simulink model "Alpha_Beta_sim"  (R2019b)
settings: Solver=VariableStepAuto  StartTime=0.0  StopTime=t_sim  FixedStep=1e-6  RelTol=1e-8  AbsTol=1e-8
values from neighbouring files (symbols this model uses):
  alphaCond = 0    [MarsTetherDynamics.m]
  betaCond = 0    [MarsTetherDynamics.m]
  dAlphaCond = 0    [MarsTetherDynamics.m]
  dBetaCond = 0    [MarsTetherDynamics.m]
  Dtheta = v/ (lt+r_hub)    (= 0.00487620861696)    [MarsTetherDynamics.m]
  g_mars = 3.71    [MarsTetherDynamics.m]
  lt = (v^2)/gamma_max    (= 824771.150189)    [MarsTetherDynamics.m]
  omega = 2*pi/T_mars    (= 7.0776580899e-05)    [MarsTetherDynamics.m]
  phi = 18.65 *pi/180    (= 0.325503905497)    [MarsTetherDynamics.m]
  r_hub = 50    [MarsTetherDynamics.m]
settings Model: Creator=valentinrichard  LastModifiedBy=valentinrichard

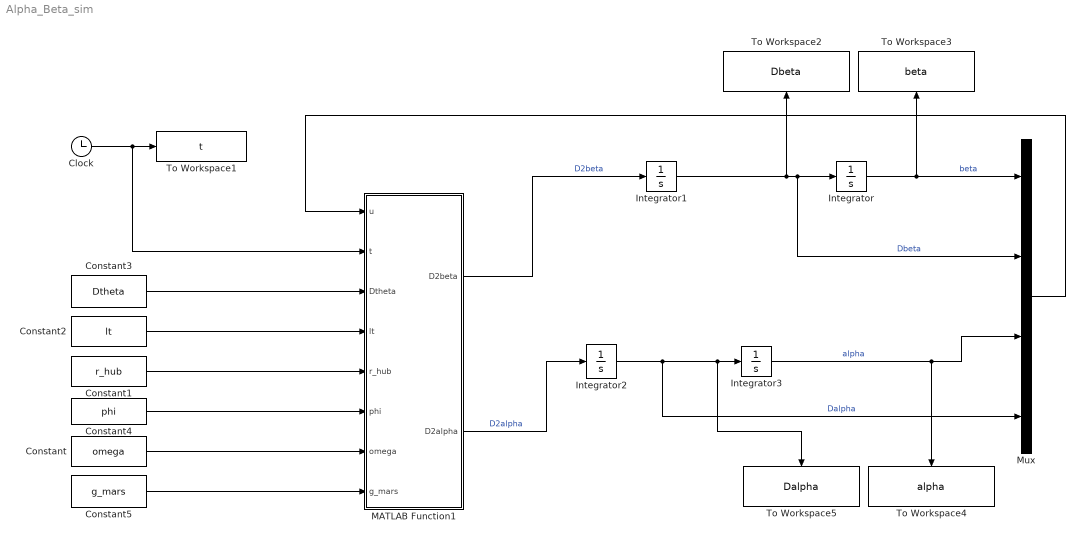
== system Alpha_Beta_sim ==
  Clock : Clock
  Constant : Constant  Value=omega
  Constant1 : Constant  Value=r_hub
  Constant2 : Constant  Value=lt
  Constant3 : Constant  Value=Dtheta
  Constant4 : Constant  Value=phi
  Constant5 : Constant  Value=g_mars
  Integrator : Integrator  InitialCondition=betaCond
  Integrator1 : Integrator  InitialCondition=dBetaCond
  Integrator2 : Integrator  InitialCondition=dAlphaCond
  Integrator3 : Integrator  InitialCondition=alphaCond
  MATLAB Function1 : MATLAB Function  TreatAsAtomicUnit=on
  Mux : Mux
  To Workspace1 : ToWorkspace  VariableName=t  SampleTime=-1
  To Workspace2 : ToWorkspace  VariableName=Dbeta  SampleTime=-1
  To Workspace3 : ToWorkspace  VariableName=beta  SampleTime=-1
  To Workspace4 : ToWorkspace  VariableName=alpha  SampleTime=-1
  To Workspace5 : ToWorkspace  VariableName=Dalpha  SampleTime=-1
  wires:
  Integrator2/1 -> To Workspace5/1, Integrator3/1, Mux/4  "Dalpha"
  Integrator1/1 -> To Workspace2/1, Mux/2, Integrator/1  "Dbeta"
  Integrator/1 -> To Workspace3/1, Mux/1  "beta"
  Integrator3/1 -> To Workspace4/1, Mux/3  "alpha"
  Mux/1 -> MATLAB Function1/1(u)
  MATLAB Function1/2(D2alpha) -> Integrator2/1  "D2alpha"
  MATLAB Function1/1(D2beta) -> Integrator1/1  "D2beta"
  Clock/1 -> MATLAB Function1/2(t), To Workspace1/1
  Constant3/1 -> MATLAB Function1/3(Dtheta)
  Constant2/1 -> MATLAB Function1/4(lt)
  Constant1/1 -> MATLAB Function1/5(r_hub)
  Constant4/1 -> MATLAB Function1/6(phi)
  Constant/1 -> MATLAB Function1/7(omega)
  Constant5/1 -> MATLAB Function1/8(g_mars)

== matlab function Alpha_Beta_sim/MATLAB Function1 ==
  data: D2beta output; u input; D2alpha output; t input; Dtheta input; lt input; r_hub input; phi input; omega input; g_mars input
function [ D2beta, D2alpha ] = ode(u,t,Dtheta,lt,r_hub,phi,omega,g_mars)
% Differential equation for Beta
%   beta = beta
%   Dbeta = d/dt (beta)
%   alpha = alpha 
%   Dalpha = d/dt (alpha)

beta = u(1);
Dbeta = u(2);
alpha = u(3);
Dalpha = u(4);


D2alpha = -2*Dbeta*tan(beta)*(Dtheta-Dalpha) ...
- r_hub*(Dtheta^2)*sin(alpha)/lt/cos(beta) ...
+ 2*omega*cos(phi)*Dbeta*(sin(Dtheta*t)*sin(alpha) + cos(Dtheta*t)*cos(alpha)) ...
- 2*omega*sin(phi)*Dbeta*tan(beta) ...
- 2*r_hub*Dtheta*omega*sin(phi)*sin(alpha)/lt/cos(beta);

D2beta = -sin(beta)*cos(beta)*(Dtheta - Dalpha)^2 ...
-r_hub*(Dtheta^2)*cos(alpha)*sin(beta)/lt ...
-g_mars*cos(beta)/lt ...
+2*omega*cos(phi)*cos(beta)^2*(Dtheta-Dalpha)*(sin(Dtheta*t)*sin(alpha)+cos(Dtheta*t)*cos(alpha)) ...
-2*omega*sin(phi)*sin(beta)*cos(beta)*(Dtheta-Dalpha) ...
+2*r_hub*omega*Dtheta*cos(Dtheta*t)*cos(phi)*cos(beta)/lt ...
-2*r_hub*omega*Dtheta*sin(phi)*cos(alpha)*sin(beta)/lt;

end
